simulink model "main_pipeline"  (R2024a)
settings: Solver=FixedStepDiscrete  StartTime=0.0  StopTime=inf  FixedStep=0.1  RelTol=1e-3
StartFcn:
  | global pipe fs
  | pipe.start();
  | 
  | for i = 1:5
  | fs = pipe.wait_for_frames();
  | end
StopFcn:
  | global pipe
  | pipe.stop();
model workspace (MATLAB code in the model file):
  | global pipe colorizer pcl_obj align_to alignedFs fs
  | global frameCount s
  | 
  | pipe = realsense.pipeline();
  | colorizer = realsense.colorizer();
  | pcl_obj = realsense.pointcloud();
  | 
  | % profile = pipe.start();
  | align_to = realsense.stream.color;
  | alignedFs = realsense.align(align_to);
  | 
  | % for i = 1:5
  | % fs = pipe.wait_for_frames();
  | % end
  | 
  | s = serial('COM3');
  | 
  | % player1 = pcplayer([-0.5 0.5],[-0.5 0.5],[0 0.5]);
  | % frameCount =0;
  | %
  | % rect = [403.51	240.51	70.98	54.98];
libraries: simulink x1, slpidlib x1
settings Model: Creator=DII_Lab  LastModifiedBy=Armando
settings SolverCC: AlgebraicLoopSolver=TrustRegion
settings DebuggingCC: UnconnectedInputMsg=warning  UnconnectedOutputMsg=warning  UnconnectedLineMsg=warning
settings ModelReferenceCC: EnableRefExpFcnMdlSchedulingChecks=on
settings SFSimCC: CustomCodeUndefinedFunction=UseInterfaceOnly
settings RTWCC: GPUComputeCapability=3.5

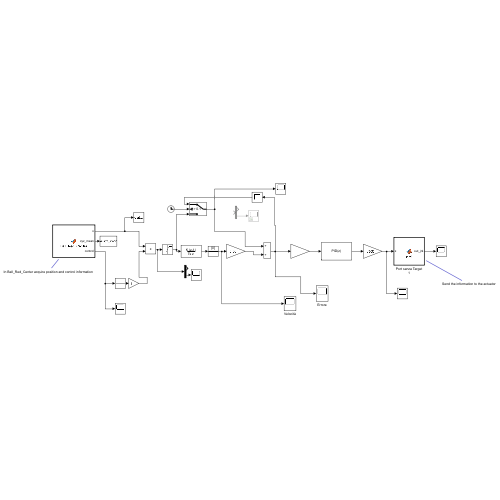
[thumbnail: Simulink's stored preview of the top-level diagram]
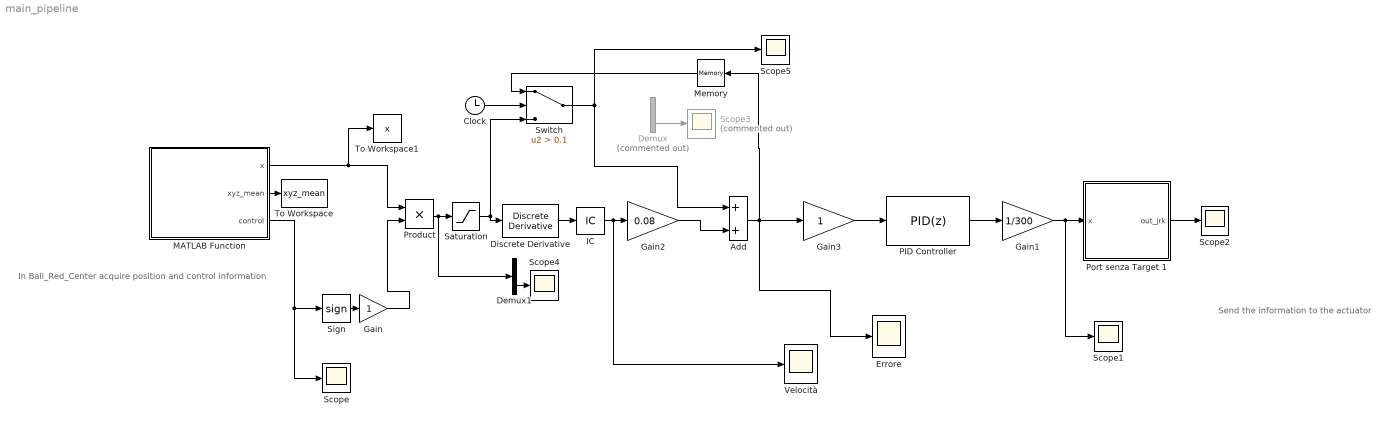
== system main_pipeline ==
  note: Send the information to the actuator
  note: In Ball_Red_Center acquire position and control information
  Add : Sum
  Clock : Clock
  Demux : Demux  Commented=on  Outputs=2
  Demux1 : Demux  Outputs=2
  Discrete Derivative : simulink/Discrete/Discrete Derivative  gainval=1  ICPrevScaledInput=0.0  OutMin=[]  OutMax=[]  OutDataType=fixdt(1, 16)  OutScaling=2^-10  DoSatur=off
  "Errore " : Scope
  Gain : Gain
  Gain1 : Gain  Gain=1/300
  Gain2 : Gain  Gain=0.08
  Gain3 : Gain
  IC : InitialCondition  Value=0
  MATLAB Function : MATLAB Function  TreatAsAtomicUnit=on
  Memory : Memory
  PID Controller : slpidlib/PID Controller  Controller=PID  Form=Parallel  TimeDomain=Discrete-time  UseExternalTs=off  SampleTime=-1  IntegratorMethod=Forward Euler  FilterMethod=Forward Euler  ControllerParametersSource=internal  P=150  I=2  UseKiTs=off  D=0  UseExternalDerivativeSource=off  N=100  UseFilter=on  TunerSelectOption=Transfer Function Based (PID Tuner App)  ZeroCross=off  InitialConditionSource=internal  InitialConditionForIntegrator=0  InitialConditionForFilter=0  DifferentiatorICPrevScaledInput=0  ExternalReset=none  TrackingMode=off  Kt=1  LimitOutput=off  SatLimitsSource=internal  UpperSaturationLimit=inf  LowerSaturationLimit=-inf  LinearizeAsGain=on  AntiWindupMode=none  Kb=1  LimitIntegrator=off  UpperIntegratorSaturationLimit=inf  LowerIntegratorSaturationLimit=-inf  POutMin=[]  POutMax=[]  IOutMin=[]  IOutMax=[]  DOutMin=[]  DOutMax=[]  NOutMin=[]  NOutMax=[]  SumOutMin=[]  SumOutMax=[]  SaturationOutMin=[]  SaturationOutMax=[]  PParamMin=[]  PParamMax=[]  IParamMin=[]  IParamMax=[]  DParamMin=[]  DParamMax=[]  NParamMin=[]  NParamMax=[]  KbParamMin=[]  KbParamMax=[]  KtParamMin=[]  KtParamMax=[]  KbOutMin=[]  KbOutMax=[]  KtOutMin=[]  KtOutMax=[]  IntegratorOutMin=[]  IntegratorOutMax=[]  FilterOutMin=[]  FilterOutMax=[]  SumI1OutMin=[]  SumI1OutMax=[]  SumI2OutMin=[]  SumI2OutMax=[]  SumI3OutMin=[]  SumI3OutMax=[]  SumI4OutMin=[]  SumI4OutMax=[]  SumDOutMin=[]  SumDOutMax=[]  DifferentiatorOutMin=[]  DifferentiatorOutMax=[]  FilterDiffOutCoefMin=[]  FilterDiffOutCoefMax=[]  ReciprocalOutMin=[]  ReciprocalOutMax=[]  SumDenOutMin=[]  SumDenOutMax=[]  SumNumOutMin=[]  SumNumOutMax=[]  DivideOutMin=[]  DivideOutMax=[]  UdiffTsProdOutMin=[]  UdiffTsProdOutMax=[]  NTsProdOutMin=[]  NTsProdOutMax=[]  UintegralTsProdOutMin=[]  UintegralTsProdOutMax=[]  UngainTsProdOutMin=[]  UngainTsProdOutMax=[]  ClampingZeroOutDataTypeStr=Inherit: Inherit via back propagation  ClampingZeroOutMin=[]  ClampingZeroOutMax=[]  FilterDenConstantOutDataTypeStr=Inherit: Inherit via back propagation  FilterDenConstantOutMin=[]  FilterDenConstantOutMax=[]  PCopyOutDataTypeStr=Inherit: Inherit via back propagation  PCopyOutMin=[]  PCopyOutMax=[]  NCopyOutDataTypeStr=Inherit: Inherit via back propagation  NCopyOutMin=[]  NCopyOutMax=[]  IntegratorContinuousStateAttributes=''  IntegratorStateMustResolveToSignalObject=off  IntegratorRTWStateStorageClass=Auto  FilterContinuousStateAttributes=''  FilterStateMustResolveToSignalObject=off  FilterRTWStateStorageClass=Auto  ParallelPVariant=InternalParameters  IdealPVariant=Disabled  IVariant=InternalParameters  DVariant=InternalParameters  IntegratorVariant=Discrete  SatVariant=Disabled  AWVariant=Passthrough  PCopyVariant=Disabled  TRVariant=Disabled  FdbkBlocksVariant=Forward  IdealPFdbkVariant=Disabled  SatFdbkVariant=Disabled  DerivativeFilterVariant=ForwardEulerFilter  NVariant=InternalParameters  NCopyVariant=Disabled  FilterICVariant=InternalICsFilter  IntegratorICVariant=InternalICs  ExternalResetVariant=Disabled  TRSumVariant=Passthrough  SumFdbkVariant=Disabled  SumVariant=Sum_PID  TsampFilterVariant=InternalTs  TsampNgainVariant=Passthrough  TsampIntegralVariant=Disabled_SignalSpec  ExternalSaturationOutDataTypeStr=Inherit: Same as second input  DerivativeSourceVariant=ErrorSignal
  Port senza Target 1 : MATLAB Function  TreatAsAtomicUnit=on
  Product : Product
  Saturation : Saturate  UpperLimit=70  LowerLimit=-70
  Scope{,1..2,4..5} (5 alike) : Scope
  Scope3 : Scope  Commented=on
  Sign : Signum
  Switch : Switch  Criteria=u2 > Threshold  Threshold=0.1  SaturateOnIntegerOverflow=off  InputSameDT=off
  To Workspace : ToWorkspace  VariableName=xyz_mean  SaveFormat=Timeseries  SampleTime=-1
  To Workspace1 : ToWorkspace  VariableName=x  SaveFormat=Timeseries  SampleTime=-1
  Velocità : Scope
  wires:
  MATLAB Function/2(xyz_mean) -> To Workspace/1
  Sign/1 -> Gain/1
  MATLAB Function/3(control) -> Sign/1, Scope/1
  Port senza Target 1/1(out_jrk) -> Scope2/1
  Gain/1 -> Product/2
  Product/1 -> Demux1/1, Saturation/1
  MATLAB Function/1(x) -> To Workspace1/1, Product/1
  Demux/2 -> Scope3/1
  Demux1/2 -> Scope4/1
  Gain1/1 -> Port senza Target 1/1(x), Scope1/1
  Discrete Derivative/1 -> IC/1
  PID Controller/1 -> Gain1/1
  Clock/1 -> Switch/2
  Switch/1 -> Add/1, Scope5/1
  Add/1 -> Memory/1, "Errore "/1, Gain3/1
  Gain2/1 -> Add/2
  IC/1 -> Velocità/1, Gain2/1
  Memory/1 -> Switch/1
  Saturation/1 -> Discrete Derivative/1, Switch/3
  Gain3/1 -> PID Controller/1

== matlab function main_pipeline/MATLAB Function ==
  data: x output; xyz_mean output; control output
function [x,xyz_mean,control]   = Ball_Red_Center

global pipe colorizer pcl_obj align_to alignedFs fs rect

%ATTENZIONE:Ricordati di cambiare gli output a tutte le funzioni quando passi da x a 
% xyz_mean

xyz_mean = zeros(1,3);

x = zeros(1,2);

control= zeros(1);


coder.extrinsic('Ball_Red_Center_F')
[x,xyz_mean,control] = Ball_Red_Center_F;

% plot3(xyz_mean(:,1), xyz_mean(:,2), xyz_mean(:,3),'rx');
% xlabel('x(m)')
% ylabel('y(m)')
% zlabel('z(m)')
% grid on
% hold on
% xyz = out.xyz_mean.Data(1,:,N_frame) %Dati sottoforma di: 1x3xN_frame
end

== matlab function main_pipeline/Port senza Target 1 ==
  data: x input; out_jrk output
function out_jrk = port(x)
% =========================================================================
% Function: port
%
% Description:
%   Sends a command to a Pololu JRK 21v3 USB motor controller through the 
%   serial port to control a linear actuator. The command is computed from 
%   an input percentage (x(2)) and converted to a JRK-compatible value.
%
% Input:
%   - x : input vector; x(2) must be a mm in [0, 100]
%
% Output:
%   - out_jrk : the scaled control value actually sent to the JRK
%
% Note:
%   - Uses hardcoded COM port ('COM3') and assumes JRK is configured to 
%     accept low-resolution target commands (0x60 and 0x61)
%   - Three control modes are available: limited excursion, oscillation, 
%     and standard control (only one should be active at a time)
%
% =========================================================================

% Allow use of non-codegen serial functionality in Simulink
coder.extrinsic('serial')

% Create serial object (update COM port as needed)
s = serial('COM3');

%% === CONTROL MODE SELECTION ===
% ⚠️ Only ONE of the following control strategies should be active

%% --- Option 1: Limited range (safe window) ---
% % Clamp input command to a range between 20% and 80%
% if x(2) > 80
%     x(2) = 80;
% elseif x(2) < 20
%     x(2) = 20;
% end

%% --- Option 2: Binary oscillation control (basic test) ---
% if x(2) >= 60
%     fopen(s)
%     fprintf(s,[170 11 97 127])  % move actuator forward
%     fclose(s)
% else
%     fopen(s)
%     fprintf(s,[170 11 96 125])  % move actuator backward
%     fclose(s)
% end

%% --- Option 3: Standard analog control ---
% Convert input mm [0–100] into JRK value range [0–4095]
out_jrk = (4095 * x(2) / 100);

% Shift to center point (JRK center = 2048)
out_jrk = 2048 - out_jrk;

% Saturate output to physical limits with ±150 margin
if out_jrk > 3000
    out_jrk = 3000;
elseif out_jrk < 1200
    out_jrk = 1200;
end

% === Command encoding and transmission ===
% JRK expects low-res target (0–255) for each direction

if out_jrk >= 0 && out_jrk <= 2048
    % Reverse direction (low half of range)
    out_cmd = fix((2048 - out_jrk) / 16);  % scale to [0–127]
    fopen(s)
    fprintf(s, [170 11 96 out_cmd])  % 0xAA, 0x0B, 0x60, value
    fclose(s)

elseif out_jrk > 2048 && out_jrk <= 4096
    % Forward direction (high half of range)
    out_cmd = fix((out_jrk - 2048) / 16);  % scale to [0–127]
    fopen(s)
    fprintf(s, [170 11 97 out_cmd])  % 0xAA, 0x0B, 0x61, value
    fclose(s)
end

end
